simulink model "fft2d"  (R2014a)
settings: Solver=FixedStepDiscrete  StartTime=0.0  StopTime=Inf  RelTol=1e-3
undefined symbols (not defined in the file): gray
libraries: visionsinks x2, visiontransforms x1, visionutilities x1, visionanalysis x1, dspvision x1
settings Model: Creator=eruffaldi  LastModifiedBy=eruffaldi

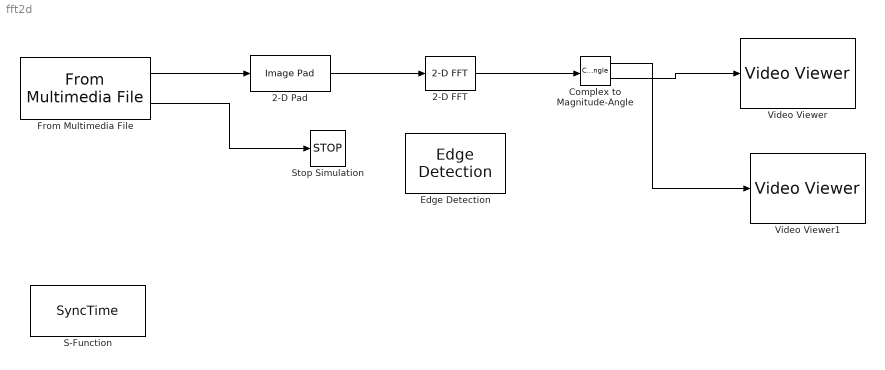
== system fft2d ==
  2-D FFT : visiontransforms/2-D FFT  TableOpt=NEW  TableOptActive=Speed  BitRevOrder=off  SkipNorm=off  FFTImplementation=Auto  firstCoeffDataTypeStr=Inherit: Same word length as input  firstCoeffLastDataTypeStr=Inherit: Same word length as input  outputMin=[]  outputMax=[]  accumDataTypeStr=Inherit: Same as product output  accumLastDataTypeStr=Inherit: Same as product output  roundingMode=Floor  overflowMode=off
  2-D Pad : visionutilities/Image Pad  method=Constant  valSrc=Specify via dialog  value=0  spec=Output size  rowDirection=Right  outRowsMode=User-specified  rowSize=2  outColSize=512  colDirection=Bottom  outColsMode=User-specified  colSize=[2 3]  outRowSize=512  trunc_flag=None
  Complex to Magnitude-Angle : ComplexToMagnitudeAngle
  Edge Detection : visionanalysis/Edge Detection  method=Sobel  outputType=Binary image  userDefinedThreshold=off  thresholdSource=Input port  threshold=20  thresholdTuning=4  edgeThinning=off  threshold_canny=[0.25 0.60]  autoPercent=70  sigma=1  prodOutputMode=Binary point scaling  prodOutputWordLength=32  prodOutputFracLength=8  roundingMode=Floor  overflowMode=off
  From Multimedia File : dspvision/From Multimedia File  inputFilename=vipboard.avi  loop=on  numPlays=inf  outputStreams=Video only  videoDataType=single  audioDataType=int16  inheritSampleTime=on  userDefinedSampleTime=1/30  noAudioOutput=off  isIntensityVideo=off  fourcc=Intensity  colorVideoFormat=Separate color signals  outputEOF=on  dataOrg=Column-major  audioFrameSize=1024  computeAudioFrameSize=off  outSamplingMode=Frame based
  S-Function : S-Function  Priority=1024  FunctionName=SyncTime  Parameters=dt  EnableBusSupport=off  mask{dt=1/30}
      mask prompts: dt "Period (s) or 0 for sleepless"
      mask Display:
      | port_label('output',1,'Unix Epoch s');
      | port_label('output',2,'Slept s');
  Stop Simulation : Stop
  Video Viewer : visionsinks/Video Viewer  inputType=Obsolete7b  imagePorts=One multidimensional signal  useColorMap=off  colormapValue=gray(256)  specRange=off  minInputVal=0  maxInputVal=255  FigPos=[681 700 410 300]  AxisZoom=on  trueSizedOnce=off  OpenAtMdlStart=on  DefaultConfigurationName=vipscopes.VideoViewerScopeCfg
  Video Viewer1 : visionsinks/Video Viewer  inputType=Obsolete7b  imagePorts=One multidimensional signal  useColorMap=off  colormapValue=gray(256)  specRange=off  minInputVal=0  maxInputVal=255  FigPos=[681 700 410 300]  AxisZoom=on  trueSizedOnce=off  OpenAtMdlStart=on  DefaultConfigurationName=vipscopes.VideoViewerScopeCfg
  wires:
  From Multimedia File/2 -> Stop Simulation/1
  From Multimedia File/1 -> 2-D Pad/1
  2-D Pad/1 -> 2-D FFT/1
  2-D FFT/1 -> Complex to Magnitude-Angle/1
  Complex to Magnitude-Angle/2 -> Video Viewer/1
  Complex to Magnitude-Angle/1 -> Video Viewer1/1
